simulink model "Gravity_Drained_Tanks_Test_WCPSv2"  (R2018a)
settings: Solver=ode45  StartTime=0.0  StopTime=10000  RelTol=1e-3  EnableMultiTasking=on
PreLoadFcn:
  | Initialize
StopFcn:
  | Plot_and_save
undefined symbols (not defined in the file or in its folder): delta_t, P
libraries: simulink x6
settings Model: Creator=tsladeche  LastModifiedBy=root
settings DataIOCC: LimitDataPoints=on  SaveFormat=Array  SignalLoggingSaveFormat=ModelDataLogs
settings OptimizationCC: ExpressionDepthLimit=2147483647  LifeSpan=inf
settings DebuggingCC: UnderspecifiedInitializationDetection=Classic  MergeDetectMultiDrivingBlocksExec=none  SolverPrmCheckMsg=warning  FcnCallInpInsideContextMsg=warning  StateNameClashWarn=warning  SFUnexpectedBacktrackingDiag=warning  SFNoUnconditionalDefaultTransitionDiag=warning  SFExecutionAtInitializationDiag=none
settings HardwareCC: ProdBitPerPointer=32  ProdBitPerSizeT=32  ProdBitPerPtrDiffT=32  ProdLargestAtomicFloat=None  ProdIntDivRoundTo=Undefined  ProdEndianess=Unspecified  ProdWordSize=32  ProdHWDeviceType=32-bit Generic
settings ModelReferenceCC: PropagateSignalLabelsOutOfModel=off
settings CodeAppCC: StateflowObjectComments=on
settings GRTTargetCC: TargetLangStandard=C89/C90 (ANSI)  GeneratePreprocessorConditionals=Disable all  CombineOutputUpdateFcns=off  GRTInterface=on
settings ConfigComp: CovMetricSettings=dw  CovHtmlReporting=on  CovSaveCumulativeToWorkspaceVar=on  CovSaveSingleToWorkspaceVar=on  CovExternalEMLEnable=off  CovSFcnEnable=off

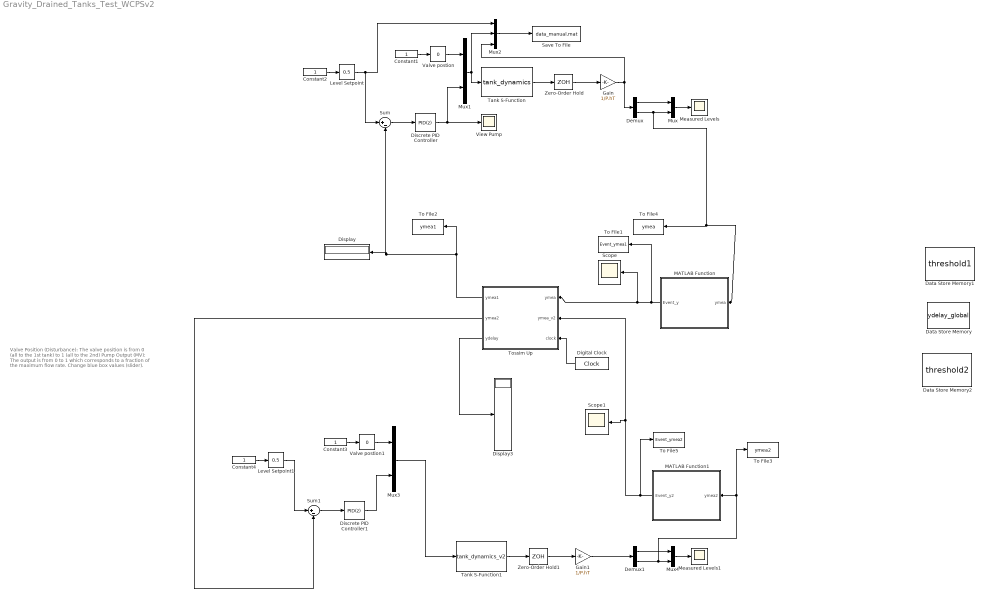
== system Gravity_Drained_Tanks_Test_WCPSv2 ==
  note: Valve Position (Disturbance): The valve position is from
      | 0 (all to the 1st tank) to 1 (all to the 2nd)
      |
      | Pump Output (MV): The output is from 0 to 1 which
      | corresponds to a fraction of the maximum flow rate.
      |
      | Change blue box values (slider).
  Constant{1..4} (4 alike) : Constant
  Data Store Memory : DataStoreMemory  DataStoreName=ydelay_global  ReadBeforeWriteMsg=warning  WriteAfterWriteMsg=warning  WriteAfterReadMsg=warning  InitialValue=[1; 1; 1; 1; 1; 1; 1; 1; 1; 1; 1; 1; 1; 1; 1]  ShowAdditionalParam=off  OutDataTypeStr=uint32
  Data Store Memory1 : DataStoreMemory  DataStoreName=threshold1  ReadBeforeWriteMsg=warning  WriteAfterWriteMsg=warning  WriteAfterReadMsg=warning  InitialValue=th1_initial  ShowAdditionalParam=off  OutDataTypeStr=double
  Data Store Memory2 : DataStoreMemory  DataStoreName=threshold2  ReadBeforeWriteMsg=warning  WriteAfterWriteMsg=warning  WriteAfterReadMsg=warning  InitialValue=th2_initial  ShowAdditionalParam=off  OutDataTypeStr=double
  Demux : Demux  Outputs=2
  Demux1 : Demux  Outputs=2
  Digital Clock : DigitalClock  SampleTime=delta_t
  Discrete PID Controller : simulink/Continuous/PID Controller  Controller=PID  TimeDomain=Discrete-time  SampleTime=delta_t  IntegratorMethod=Forward Euler  FilterMethod=Forward Euler  Form=Parallel  UseFilter=on  ControllerParametersSource=internal  P=1/1.624181124  I=(1/1.624181124)/140.7309944  D=0  N=100  InitialConditionSource=internal  InitialConditionForIntegrator=0  InitialConditionForFilter=0  ExternalReset=none  LimitOutput=on  UpperSaturationLimit=1  LowerSaturationLimit=0  LinearizeAsGain=on  AntiWindupMode=clamping  Kb=1  TrackingMode=off  Kt=1  PParamMin=[]  PParamMax=[]  IParamMin=[]  IParamMax=[]  DParamMin=[]  DParamMax=[]  NParamMin=[]  NParamMax=[]  KbParamMin=[]  KbParamMax=[]  KtParamMin=[]  KtParamMax=[]  POutMin=[]  POutMax=[]  IOutMin=[]  IOutMax=[]  DOutMin=[]  DOutMax=[]  NOutMin=[]  NOutMax=[]  KbOutMin=[]  KbOutMax=[]  KtOutMin=[]  KtOutMax=[]  IntegratorOutMin=[]  IntegratorOutMax=[]  FilterOutMin=[]  FilterOutMax=[]  SumOutMin=[]  SumOutMax=[]  SumI1OutMin=[]  SumI1OutMax=[]  SumI2OutMin=[]  SumI2OutMax=[]  SumI3OutMin=[]  SumI3OutMax=[]  SumDOutMin=[]  SumDOutMax=[]  SaturationOutMin=[]  SaturationOutMax=[]  IntegratorContinuousStateAttributes=''  IntegratorStateMustResolveToSignalObject=off  IntegratorRTWStateStorageClass=Auto  FilterContinuousStateAttributes=''  FilterStateMustResolveToSignalObject=off  FilterRTWStateStorageClass=Auto  DifferentiatorICPrevScaledInput=0  DifferentiatorOutMin=[]  DifferentiatorOutMax=[]  FilterDiffOutCoefMin=[]  FilterDiffOutCoefMax=[]  SumDenOutMin=[]  SumDenOutMax=[]  SumNumOutMin=[]  SumNumOutMax=[]  ReciprocalOutMin=[]  ReciprocalOutMax=[]  DivideOutMin=[]  DivideOutMax=[]  TunerSelectOption=Transfer Function Based (PID Tuner App)
  Discrete PID Controller1 : simulink/Continuous/PID Controller  Controller=PID  TimeDomain=Discrete-time  SampleTime=delta_t  IntegratorMethod=Forward Euler  FilterMethod=Forward Euler  Form=Parallel  UseFilter=on  ControllerParametersSource=internal  P=1/1.624181124  I=(1/1.624181124)/140.7309944  D=0  N=100  InitialConditionSource=internal  InitialConditionForIntegrator=0  InitialConditionForFilter=0  ExternalReset=none  LimitOutput=on  UpperSaturationLimit=1  LowerSaturationLimit=0  LinearizeAsGain=on  AntiWindupMode=clamping  Kb=1  TrackingMode=off  Kt=1  PParamMin=[]  PParamMax=[]  IParamMin=[]  IParamMax=[]  DParamMin=[]  DParamMax=[]  NParamMin=[]  NParamMax=[]  KbParamMin=[]  KbParamMax=[]  KtParamMin=[]  KtParamMax=[]  POutMin=[]  POutMax=[]  IOutMin=[]  IOutMax=[]  DOutMin=[]  DOutMax=[]  NOutMin=[]  NOutMax=[]  KbOutMin=[]  KbOutMax=[]  KtOutMin=[]  KtOutMax=[]  IntegratorOutMin=[]  IntegratorOutMax=[]  FilterOutMin=[]  FilterOutMax=[]  SumOutMin=[]  SumOutMax=[]  SumI1OutMin=[]  SumI1OutMax=[]  SumI2OutMin=[]  SumI2OutMax=[]  SumI3OutMin=[]  SumI3OutMax=[]  SumDOutMin=[]  SumDOutMax=[]  SaturationOutMin=[]  SaturationOutMax=[]  IntegratorContinuousStateAttributes=''  IntegratorStateMustResolveToSignalObject=off  IntegratorRTWStateStorageClass=Auto  FilterContinuousStateAttributes=''  FilterStateMustResolveToSignalObject=off  FilterRTWStateStorageClass=Auto  DifferentiatorICPrevScaledInput=0  DifferentiatorOutMin=[]  DifferentiatorOutMax=[]  FilterDiffOutCoefMin=[]  FilterDiffOutCoefMax=[]  SumDenOutMin=[]  SumDenOutMax=[]  SumNumOutMin=[]  SumNumOutMax=[]  ReciprocalOutMin=[]  ReciprocalOutMax=[]  DivideOutMin=[]  DivideOutMax=[]  TunerSelectOption=Transfer Function Based (PID Tuner App)
  Display : Display
  Display3 : Display
  Gain : Gain  Gain=1/P.hT
  Gain1 : Gain  Gain=1/P.hT
  Level Setpoint : simulink/Math Operations/Slider Gain  gain=0.5  low=0  high=1
  Level Setpoint1 : simulink/Math Operations/Slider Gain  gain=0.5  low=0  high=1
  MATLAB Function : MATLAB Function  TreatAsAtomicUnit=on
  MATLAB Function1 : MATLAB Function  TreatAsAtomicUnit=on
  Measured Levels : Scope
  Measured Levels1 : Scope
  Mux{,1,3..4} (4 alike) : Mux  Inputs=2
  Mux2 : Mux  Inputs=3
  Save To File : ToFile  Filename=data_manual.mat  MatrixName=tanks  SampleTime=delta_t
  Scope : Scope
  Scope1 : Scope
  Sum : Sum  Inputs=|+-
  Sum1 : Sum  Inputs=|+-
  Tank S-Function : S-Function  FunctionName=tank_dynamics  Parameters=P  SFunctionDeploymentMode=off  EnableBusSupport=off
  Tank S-Function1 : S-Function  FunctionName=tank_dynamics_v2  Parameters=P  SFunctionDeploymentMode=off  EnableBusSupport=off
  To File1 : ToFile  Filename=Event_ymea1  MatrixName=Event_ymea1  SampleTime=1
  To File2 : ToFile  Filename=ymea1  MatrixName=ymea1  SampleTime=1
  To File3 : ToFile  Filename=ymea2  MatrixName=ymea2  SampleTime=1
  To File4 : ToFile  Filename=ymea  MatrixName=ymea  SampleTime=1
  To File5 : ToFile  Filename=Event_ymea2  MatrixName=Event_ymea2  SampleTime=1
  Tossim Up : MATLAB Function  TreatAsAtomicUnit=on
  Valve postion : simulink/Math Operations/Slider Gain  gain=0  low=0  high=1
  Valve postion1 : simulink/Math Operations/Slider Gain  gain=0  low=0  high=1
  View Pump : Scope
  Zero-Order Hold : ZeroOrderHold  SampleTime=delta_t
  Zero-Order Hold1 : ZeroOrderHold  SampleTime=delta_t
  wires:
  Gain/1 -> Demux/1, Mux2/3
  Mux2/1 -> Save To File/1
  Constant1/1 -> Valve postion/1
  Mux1/1 -> Mux2/2, Tank S-Function/1
  Valve postion/1 -> Mux1/1
  Constant2/1 -> Level Setpoint/1
  Level Setpoint/1 -> Sum/1, Mux2/1
  Mux/1 -> Measured Levels/1
  Demux/1 -> Mux/1
  Demux/2 -> MATLAB Function/1(ymea), To File4/1, Mux/2
  Sum/1 -> Discrete PID Controller/1
  Discrete PID Controller/1 -> Mux1/2, View Pump/1
  Tank S-Function/1 -> Zero-Order Hold/1
  Zero-Order Hold/1 -> Gain/1
  Tossim Up/1(ymea1) -> To File2/1, Display/1, Sum/2
  Tossim Up/3(ydelay) -> Display3/1
  Level Setpoint1/1 -> Sum1/1
  Valve postion1/1 -> Mux3/1
  Discrete PID Controller1/1 -> Mux3/2
  Mux3/1 -> Tank S-Function1/1
  Constant3/1 -> Valve postion1/1
  Constant4/1 -> Level Setpoint1/1
  Sum1/1 -> Discrete PID Controller1/1
  Tank S-Function1/1 -> Zero-Order Hold1/1
  Zero-Order Hold1/1 -> Gain1/1
  Mux4/1 -> Measured Levels1/1
  Demux1/1 -> Mux4/1
  Gain1/1 -> Demux1/1
  Demux1/2 -> MATLAB Function1/1(ymea2), To File3/1, Mux4/2
  Tossim Up/2(ymea2) -> Sum1/2
  MATLAB Function/1(Event_y) -> To File1/1, Scope/1, Tossim Up/1(ymea)
  MATLAB Function1/1(Event_y2) -> To File5/1, Scope1/1, Tossim Up/2(ymea_v2)
  Digital Clock/1 -> Tossim Up/3(clock)

== matlab function Gravity_Drained_Tanks_Test_WCPSv2/Tossim Up ==
  settings: updateMethod=DISCRETE
  data: ymea1 output; ymea2 output; ymea input; ydelay output; ydelay_global data_store_memory; ymea_v2 input; clock input
function [ymea1,ymea2, ydelay]  = Tossim_block(ymea, ymea_v2, clock)
% Inputs:
% ymea: measurement from structure
% Outputs:
% ymea1: measurement output
% ydelay: delay traces
persistent delay1 past_ymea csi_ydelay past_ymea_v2% delay trace
persistent i Task_period % count 
global ydelay_global 


% allow these matlab functions to be used in Embedded Matlab block
eml.extrinsic('python');
eml.extrinsic('num2str');
eml.extrinsic('str2num');
eml.extrinsic('delay_summary');
eml.extrinsic('disp');
eml.extrinsic('ps_aggregation');
eml.extrinsic('for');
eml.extrinsic('end');

if isempty(i)
    i = 0;
    %past_ymea = 0;
    past_ymea = ymea;
    past_ymea_v2 = ymea_v2;
    csi_ydelay = past_ymea;
    Task_period = [10 10 4];        %Task_period=[10 10 4] * 10
end

%[row column] = size(Task_period_time);

ydelay = [1 0 0 0 0 0 0 0 0]';
% call python to communicate with TOSSIM

call_count = 1; %Superframelength
rssi = -69;%sensor rssi

[resultz] = ps_aggregation(call_count, rssi);%here call TOSSIM Client ----yh
end_to_end_delivery_result_aggregated = sum(resultz)

resultz

%[delay] = delay_summary(end_to_end_delivery_result_aggregated);
[delay] = delay_summary(resultz);

delay

% for event trigger!!!
Task_period_time = Task_period * 10;
for j=Task_period_time(1,1:end)
    if(rem(clock,j) == 0)
        if(j == Task_period_time(1,1))      %Need to revise when # of Task is changed
           past_ymea = ymea;
        elseif(j == Task_period_time(1,2))
            past_ymea_v2 = ymea_v2;
        end
    end
end


ydelay = delay';

delay1 = ydelay;
x =ydelay(2);
i = i+1;

%ymea1 = ymea;

for i_yg = 1:9
    ydelay_global(i_yg, 1) = ydelay(i_yg, 1);
end
delay = ydelay';

ymea_v1_index = 1;
ymea_v2_index = 2;
if delay(1,ymea_v1_index + 1)~=88
    %csi_ydelay = past_ymea;
    ymea1 = past_ymea;
    past_ymea = ymea;
    %%%%
    ymea2 = past_ymea_v2;
elseif delay(1,ymea_v2_index + 1)~=88
    ymea2 = past_ymea_v2;
    past_ymea_v2 = ymea_v2;
    %%%
    ymea1 = past_ymea;
else
    ymea1 = past_ymea;
    ymea2 = past_ymea_v2;
end

== matlab function Gravity_Drained_Tanks_Test_WCPSv2/MATLAB Function ==
  data: ymea input; Event_y output; threshold1 data_store_memory
function Event_y = event_trigger(ymea)

persistent previous_ymea
persistent i %count
global threshold1


if isempty(i)
    i = 0;
    previous_ymea = 0;
end

compare = abs(ymea - previous_ymea);
if (compare) >= threshold1
    ans = ymea;
    previous_ymea = ymea;
else
    ans = previous_ymea;
end

i = i + 1;
Event_y = ans;

== matlab function Gravity_Drained_Tanks_Test_WCPSv2/MATLAB Function1 ==
  data: ymea2 input; Event_y2 output; threshold2 data_store_memory
function Event_y2 = event_trigger2(ymea2)

persistent previous_ymea
persistent i %count
global threshold2


if isempty(i)
    i = 0;
    previous_ymea = 0;
end

compare = abs(ymea2 - previous_ymea);
if (compare) >= threshold2
    ans = ymea2;
    previous_ymea = ymea2;
else
    ans = previous_ymea;
end

i = i + 1;
Event_y2 = ans;
